simulink library "inp"  (R2021b)
settings: Solver=VariableStepAuto  StartTime=0.0  StopTime=10.0  RelTol=1e-3
undefined symbols (not defined in the file): C_TASK_5MS_S, FALSE, KINP_AcoreReadyToSlp_flg_ovrdflg, KINP_AcoreReadyToSlp_flg_ovrdval, KINP_AllowMovThd_OTA_enum_ovrdflg, KINP_AllowMovThd_OTA_enum_ovrdval, KINP_APSAngleTarget_Deg_ovrdflg, KINP_APSAngleTarget_Deg_ovrdval, KINP_APSDecReq_mps2_ovrdflg, KINP_APSDecReq_mps2_ovrdval, KINP_APSDecReqA_flg_ovrdflg, KINP_APSDecReqA_flg_ovrdval, KINP_APSDFLL_cm_ovrdflg, KINP_APSDFLL_cm_ovrdval, KINP_APSDFLR_cm_ovrdflg, KINP_APSDFLR_cm_ovrdval, KINP_APSDRLL_cm_ovrdflg, KINP_APSDRLL_cm_ovrdval, KINP_APSDRLR_cm_ovrdflg, KINP_APSDRLR_cm_ovrdval, KINP_APSExitCondition_enum_ovrdflg, KINP_APSExitCondition_enum_ovrdval, KINP_APSHWVer_enum_ovrdflg, KINP_APSHWVer_enum_ovrdval, KINP_APSProgressPCT_pct_ovrdflg, KINP_APSProgressPCT_pct_ovrdval, KINP_APSReq_enum_ovrdflg, KINP_APSReq_enum_ovrdval, KINP_APSRQDisplay_enum_ovrdflg, KINP_APSRQDisplay_enum_ovrdval, KINP_APSRqEPASCtrl_flg_ovrdflg, KINP_APSRqEPASCtrl_flg_ovrdval, KINP_APSShiftPosnReq_enum_ovrdval, KINP_APSShiftPosnReq_enum_ovrflg, KINP_APSSpeedCMD_kph_ovrdval, KINP_APSSpeedCMD_kph_ovrflg, KINP_APSStaSystem_enum_ovrdflg, KINP_APSStaSystem_enum_ovrdval, KINP_APSSWVer_enum_ovrdflg, KINP_APSSWVer_enum_ovrdval, KINP_APSVMCReqA_flg_ovrdval, KINP_APSVMCReqA_flg_ovrflg, KINP_APSVRqEPASCtrl_flg_ovrdflg, KINP_APSVRqEPASCtrl_flg_ovrdval, KINP_AuxBattVolmV_mV_ovrdflg, KINP_AuxBattVolmV_mV_ovrdval, KINP_CAASSta_enum_ovrdflg, KINP_CAASSta_enum_ovrdval, KINP_CAASVMCReqA_flg_ovrdval, KINP_CAASVMCReqA_flg_ovrflg, KINP_Chime_enum_ovrdflg, KINP_Chime_enum_ovrdval, KINP_ClearDTCcmd_flg_ovrdflg, KINP_ClearDTCcmd_flg_ovrdval, KINP_EvccAplusPwrUpReq_flg_ovrdflg, KINP_EvccAplusPwrUpReq_flg_ovrdval, KINP_LFID_raw_ovrdval, KINP_LFID_raw_ovrflg, KINP_LRID_raw_ovrdval, KINP_MemOffsetAccX_raw16_ovrdflg ... (+118)
libraries: FVT_lib x595, hcu_lib x1
(part 8 of 27)

== system inp/INP/GPIO/Digital ==
  BHAL_outputs : Inport
  BrakeLampSW : FVT_lib/inp/di_signal_template  SystemSampleTime=-1  VariantActivationTime=update diagram  Latency=0  AutoFrameSizeCalculation=off
      link override debdec: Value=KINP_BrakeLampSW_flg_debdec
      link override debinc: Value=KINP_BrakeLampSW_flg_debinc
      link override deblim: Value=KINP_BrakeLampSW_flg_deblim
      link override inverse: Value=KINP_BrakeLampSW_flg_inverse
      link override ovrdflg: Value=KINP_BrakeLampSW_flg_ovrdflg
      link override ovrdval: Value=KINP_BrakeLampSW_flg_ovrdval
      link override srvcflg: Value=KINP_BrakeLampSW_flg_srvcflg
      link override srvcval: Value=KINP_BrakeLampSW_flg_srvcval
  BrakeSWGPIO : FVT_lib/inp/di_signal_template  SystemSampleTime=-1  VariantActivationTime=update diagram  Latency=0  AutoFrameSizeCalculation=off
      link override debdec: Value=KINP_BrakeSWGPIO_flg_debdec
      link override debinc: Value=KINP_BrakeSWGPIO_flg_debinc
      link override deblim: Value=KINP_BrakeSWGPIO_flg_deblim
      link override inverse: Value=KINP_BrakeSWGPIO_flg_inverse
      link override ovrdflg: Value=KINP_BrakeSWGPIO_flg_ovrdflg
      link override ovrdval: Value=KINP_BrakeSWGPIO_flg_ovrdval
      link override srvcflg: Value=KINP_BrakeSWGPIO_flg_srvcflg
      link override srvcval: Value=KINP_BrakeSWGPIO_flg_srvcval
  CentralDoorLockSW : FVT_lib/inp/di_signal_template  SystemSampleTime=-1  VariantActivationTime=update diagram  Latency=0  AutoFrameSizeCalculation=off
      link override debdec: Value=KINP_CentralDoorLockSW_flg_debdec
      link override debinc: Value=KINP_CentralDoorLockSW_flg_debinc
      link override deblim: Value=KINP_CentralDoorLockSW_flg_deblim
      link override inverse: Value=KINP_CentralDoorLockSW_flg_inverse
      link override ovrdflg: Value=KINP_CentralDoorLockSW_flg_ovrdflg
      link override ovrdval: Value=KINP_CentralDoorLockSW_flg_ovrdval
      link override srvcflg: Value=KINP_CentralDoorLockSW_flg_srvcflg
      link override srvcval: Value=KINP_CentralDoorLockSW_flg_srvcval
  CrashSignalGPIO : FVT_lib/inp/di_signal_template  SystemSampleTime=-1  VariantActivationTime=update diagram  Latency=0  AutoFrameSizeCalculation=off
      link override debdec: Value=KINP_CrashSignalGPIO_flg_debdec
      link override debinc: Value=KINP_CrashSignalGPIO_flg_debinc
      link override deblim: Value=KINP_CrashSignalGPIO_flg_deblim
      link override inverse: Value=KINP_CrashSignalGPIO_flg_inverse
      link override ovrdflg: Value=KINP_CrashSignalGPIO_flg_ovrdflg
      link override ovrdval: Value=KINP_CrashSignalGPIO_flg_ovrdval
      link override srvcflg: Value=KINP_CrashSignalGPIO_flg_srvcflg
      link override srvcval: Value=KINP_CrashSignalGPIO_flg_srvcval
  DrDoorSW : FVT_lib/inp/di_signal_template  SystemSampleTime=-1  VariantActivationTime=update diagram  Latency=0  AutoFrameSizeCalculation=off
      link override debdec: Value=KINP_DrDoorSW_flg_debdec
      link override debinc: Value=KINP_DrDoorSW_flg_debinc
      link override deblim: Value=KINP_DrDoorSW_flg_deblim
      link override inverse: Value=KINP_DrDoorSW_flg_inverse
      link override ovrdflg: Value=KINP_DrDoorSW_flg_ovrdflg
      link override ovrdval: Value=KINP_DrDoorSW_flg_ovrdval
      link override srvcflg: Value=KINP_DrDoorSW_flg_srvcflg
      link override srvcval: Value=KINP_DrDoorSW_flg_srvcval
  HazardSW : FVT_lib/inp/di_signal_template  SystemSampleTime=-1  VariantActivationTime=update diagram  Latency=0  AutoFrameSizeCalculation=off
      link override debdec: Value=KINP_HazardSW_flg_debdec
      link override debinc: Value=KINP_HazardSW_flg_debinc
      link override deblim: Value=KINP_HazardSW_flg_deblim
      link override inverse: Value=KINP_HazardSW_flg_inverse
      link override ovrdflg: Value=KINP_HazardSW_flg_ovrdflg
      link override ovrdval: Value=KINP_HazardSW_flg_ovrdval
      link override srvcflg: Value=KINP_HazardSW_flg_srvcflg
      link override srvcval: Value=KINP_HazardSW_flg_srvcval
  HoodSW : FVT_lib/inp/di_signal_template  SystemSampleTime=-1  VariantActivationTime=update diagram  Latency=0  AutoFrameSizeCalculation=off
      link override debdec: Value=KINP_HoodSW_flg_debdec
      link override debinc: Value=KINP_HoodSW_flg_debinc
      link override deblim: Value=KINP_HoodSW_flg_deblim
      link override inverse: Value=KINP_HoodSW_flg_inverse
      link override ovrdflg: Value=KINP_HoodSW_flg_ovrdflg
      link override ovrdval: Value=KINP_HoodSW_flg_ovrdval
      link override srvcflg: Value=KINP_HoodSW_flg_srvcflg
      link override srvcval: Value=KINP_HoodSW_flg_srvcval
  PsDoorSW : FVT_lib/inp/di_signal_template  SystemSampleTime=-1  VariantActivationTime=update diagram  Latency=0  AutoFrameSizeCalculation=off
      link override debdec: Value=KINP_PsDoorSW_flg_debdec
      link override debinc: Value=KINP_PsDoorSW_flg_debinc
      link override deblim: Value=KINP_PsDoorSW_flg_deblim
      link override inverse: Value=KINP_PsDoorSW_flg_inverse
      link override ovrdflg: Value=KINP_PsDoorSW_flg_ovrdflg
      link override ovrdval: Value=KINP_PsDoorSW_flg_ovrdval
      link override srvcflg: Value=KINP_PsDoorSW_flg_srvcflg
      link override srvcval: Value=KINP_PsDoorSW_flg_srvcval
  RLDoorSW : FVT_lib/inp/di_signal_template  SystemSampleTime=-1  VariantActivationTime=update diagram  Latency=0  AutoFrameSizeCalculation=off
      link override debdec: Value=KINP_RLDoorSW_flg_debdec
      link override debinc: Value=KINP_RLDoorSW_flg_debinc
      link override deblim: Value=KINP_RLDoorSW_flg_deblim
      link override inverse: Value=KINP_RLDoorSW_flg_inverse
      link override ovrdflg: Value=KINP_RLDoorSW_flg_ovrdflg
      link override ovrdval: Value=KINP_RLDoorSW_flg_ovrdval
      link override srvcflg: Value=KINP_RLDoorSW_flg_srvcflg
      link override srvcval: Value=KINP_RLDoorSW_flg_srvcval
  RRDoorSW : FVT_lib/inp/di_signal_template  SystemSampleTime=-1  VariantActivationTime=update diagram  Latency=0  AutoFrameSizeCalculation=off
      link override debdec: Value=KINP_RRDoorSW_flg_debdec
      link override debinc: Value=KINP_RRDoorSW_flg_debinc
      link override deblim: Value=KINP_RRDoorSW_flg_deblim
      link override inverse: Value=KINP_RRDoorSW_flg_inverse
      link override ovrdflg: Value=KINP_RRDoorSW_flg_ovrdflg
      link override ovrdval: Value=KINP_RRDoorSW_flg_ovrdval
      link override srvcflg: Value=KINP_RRDoorSW_flg_srvcflg
      link override srvcval: Value=KINP_RRDoorSW_flg_srvcval
  SeatSW : FVT_lib/inp/di_signal_template  SystemSampleTime=-1  VariantActivationTime=update diagram  Latency=0  AutoFrameSizeCalculation=off
      link override debdec: Value=KINP_SeatSW_flg_debdec
      link override debinc: Value=KINP_SeatSW_flg_debinc
      link override deblim: Value=KINP_SeatSW_flg_deblim
      link override inverse: Value=KINP_SeatSW_flg_inverse
      link override ovrdflg: Value=KINP_SeatSW_flg_ovrdflg
      link override ovrdval: Value=KINP_SeatSW_flg_ovrdval
      link override srvcflg: Value=KINP_SeatSW_flg_srvcflg
      link override srvcval: Value=KINP_SeatSW_flg_srvcval
  TailgateSW : FVT_lib/inp/di_signal_template  SystemSampleTime=-1  VariantActivationTime=update diagram  Latency=0  AutoFrameSizeCalculation=off
      link override debdec: Value=KINP_TailgateSW_flg_debdec
      link override debinc: Value=KINP_TailgateSW_flg_debinc
      link override deblim: Value=KINP_TailgateSW_flg_deblim
      link override inverse: Value=KINP_TailgateSW_flg_inverse
      link override ovrdflg: Value=KINP_TailgateSW_flg_ovrdflg
      link override ovrdval: Value=KINP_TailgateSW_flg_ovrdval
      link override srvcflg: Value=KINP_TailgateSW_flg_srvcflg
      link override srvcval: Value=KINP_TailgateSW_flg_srvcval
  TrunkHanSW : FVT_lib/inp/di_signal_template  SystemSampleTime=-1  VariantActivationTime=update diagram  Latency=0  AutoFrameSizeCalculation=off
      link override debdec: Value=KINP_TrunkHanSW_flg_debdec
      link override debinc: Value=KINP_TrunkHanSW_flg_debinc
      link override deblim: Value=KINP_TrunkHanSW_flg_deblim
      link override inverse: Value=KINP_TrunkHanSW_flg_inverse
      link override ovrdflg: Value=KINP_TrunkHanSW_flg_ovrdflg
      link override ovrdval: Value=KINP_TrunkHanSW_flg_ovrdval
      link override srvcflg: Value=KINP_TrunkHanSW_flg_srvcflg
      link override srvcval: Value=KINP_TrunkHanSW_flg_srvcval
  slr_VINP_BrakeLampSW_flg : BusSelector  OutputSignals=VHAL_BrakeLampSW_flg
  slr_VINP_BrakeSWGPIO_flg : BusSelector  OutputSignals=VHAL_BrakeSWGPIO_flg
  slr_VINP_CentralDoorLockSW_flg : BusSelector  OutputSignals=VHAL_CentralDoorLockSW_flg
  slr_VINP_CrashSignalGPIO_flg : BusSelector  OutputSignals=VHAL_CrashSignalGPIO_flg
  slr_VINP_DrDoorSW_flg : BusSelector  OutputSignals=VHAL_DrDoorSW_flg
  slr_VINP_HazardSW_flg : BusSelector  OutputSignals=VHAL_HazardSW_flg
  slr_VINP_HoodSW_flg : BusSelector  OutputSignals=VHAL_HoodSW_flg
  slr_VINP_PsDoorSW_flg : BusSelector  OutputSignals=VHAL_PsDoorSW_flg
  slr_VINP_RLDoorSW_flg : BusSelector  OutputSignals=VHAL_RLDoorSW_flg
  slr_VINP_RRDoorSW_flg : BusSelector  OutputSignals=VHAL_RRDoorSW_flg
  slr_VINP_SeatSW_flg : BusSelector  OutputSignals=VHAL_SeatSW_flg
  slr_VINP_TailgateSW_flg : BusSelector  OutputSignals=VHAL_TailgateSW_flg
  slr_VINP_TrunkHanSW_flg : BusSelector  OutputSignals=VHAL_TrunkHanSW_flg
  VINP_BrakeSWGPIO_flg : Outport
  VINP_HoodSW_flg : Outport  Port=2
  VINP_TailgateSW_flg : Outport  Port=3
  VINP_DrDoorSW_flg : Outport  Port=4
  VINP_PsDoorSW_flg : Outport  Port=5
  VINP_RRDoorSW_flg : Outport  Port=6
  VINP_RLDoorSW_flg : Outport  Port=7
  VINP_CentralDoorLockSW_flg : Outport  Port=8
  VINP_HazardSW_flg : Outport  Port=9
  VINP_BrakeLampSW_flg : Outport  Port=10
  VINP_TrunkHanSW_flg : Outport  Port=11
  VINP_SeatSW_flg : Outport  Port=12
  VINP_CrashSignalGPIO_flg : Outport  Port=13
  wires:
  BHAL_outputs/1 -> [BHAL_outputs]
  BrakeSWGPIO/1 -> VINP_BrakeSWGPIO_flg/1  "VINP_BrakeSWGPIO_flg"
  [BHAL_outputs] -> slr_VINP_BrakeSWGPIO_flg/1
  slr_VINP_BrakeSWGPIO_flg/1 -> BrakeSWGPIO/1  "<VHAL_BrakeSWGPIO_flg>"
  HoodSW/1 -> VINP_HoodSW_flg/1  "VINP_HoodSW_flg"
  [BHAL_outputs] -> slr_VINP_HoodSW_flg/1
  slr_VINP_HoodSW_flg/1 -> HoodSW/1  "<VHAL_HoodSW_flg>"
  TailgateSW/1 -> VINP_TailgateSW_flg/1  "VINP_TailgateSW_flg"
  [BHAL_outputs] -> slr_VINP_TailgateSW_flg/1
  slr_VINP_TailgateSW_flg/1 -> TailgateSW/1  "<VHAL_TailgateSW_flg>"
  DrDoorSW/1 -> VINP_DrDoorSW_flg/1  "VINP_DrDoorSW_flg"
  [BHAL_outputs] -> slr_VINP_DrDoorSW_flg/1
  slr_VINP_DrDoorSW_flg/1 -> DrDoorSW/1  "<VHAL_DrDoorSW_flg>"
  PsDoorSW/1 -> VINP_PsDoorSW_flg/1  "VINP_PsDoorSW_flg"
  [BHAL_outputs] -> slr_VINP_PsDoorSW_flg/1
  slr_VINP_PsDoorSW_flg/1 -> PsDoorSW/1  "<VHAL_PsDoorSW_flg>"
  RRDoorSW/1 -> VINP_RRDoorSW_flg/1  "VINP_RRDoorSW_flg"
  [BHAL_outputs] -> slr_VINP_RRDoorSW_flg/1
  slr_VINP_RRDoorSW_flg/1 -> RRDoorSW/1  "<VHAL_RRDoorSW_flg>"
  RLDoorSW/1 -> VINP_RLDoorSW_flg/1  "VINP_RLDoorSW_flg"
  [BHAL_outputs] -> slr_VINP_RLDoorSW_flg/1
  slr_VINP_RLDoorSW_flg/1 -> RLDoorSW/1  "<VHAL_RLDoorSW_flg>"
  CentralDoorLockSW/1 -> VINP_CentralDoorLockSW_flg/1  "VINP_CentralDoorLockSW_flg"
  [BHAL_outputs] -> slr_VINP_CentralDoorLockSW_flg/1
  slr_VINP_CentralDoorLockSW_flg/1 -> CentralDoorLockSW/1  "<VHAL_CentralDoorLockSW_flg>"
  HazardSW/1 -> VINP_HazardSW_flg/1  "VINP_HazardSW_flg"
  [BHAL_outputs] -> slr_VINP_HazardSW_flg/1
  slr_VINP_HazardSW_flg/1 -> HazardSW/1  "<VHAL_HazardSW_flg>"
  BrakeLampSW/1 -> VINP_BrakeLampSW_flg/1  "VINP_BrakeLampSW_flg"
  [BHAL_outputs] -> slr_VINP_BrakeLampSW_flg/1
  slr_VINP_BrakeLampSW_flg/1 -> BrakeLampSW/1  "<VHAL_BrakeLampSW_flg>"
  TrunkHanSW/1 -> VINP_TrunkHanSW_flg/1  "VINP_TrunkHanSW_flg"
  [BHAL_outputs] -> slr_VINP_TrunkHanSW_flg/1
  slr_VINP_TrunkHanSW_flg/1 -> TrunkHanSW/1  "<VHAL_TrunkHanSW_flg>"
  SeatSW/1 -> VINP_SeatSW_flg/1  "VINP_SeatSW_flg"
  [BHAL_outputs] -> slr_VINP_SeatSW_flg/1
  slr_VINP_SeatSW_flg/1 -> SeatSW/1  "<VHAL_SeatSW_flg>"
  [BHAL_outputs] -> slr_VINP_CrashSignalGPIO_flg/1
  slr_VINP_CrashSignalGPIO_flg/1 -> CrashSignalGPIO/1  "<VHAL_CrashSignalGPIO_flg>"
  CrashSignalGPIO/1 -> VINP_CrashSignalGPIO_flg/1  "VINP_CrashSignalGPIO_flg"

== system inp/INP/IMU/Subsystem1 ==
  In1 : Inport
  Constant : Constant  Value=KINP_MemOffsetGyroY_raw16_ovrdval
  Constant1 : Constant  Value=KINP_MemOffsetGyroY_raw16_ovrdflg
  Switch : Switch  Criteria=u2 ~= 0
  Out1 : Outport
  wires:
  Switch/1 -> Out1/1
  Constant/1 -> Switch/1
  Constant1/1 -> Switch/2
  In1/1 -> Switch/3

== system inp/INP/IMU/Subsystem10 ==
  In1 : Inport
  Constant : Constant  Value=KINP_SensingAccZ_raw16_ovrdval
  Constant1 : Constant  Value=KINP_SensingAccZ_raw16_ovrdflg
  Switch : Switch  Criteria=u2 ~= 0
  Out1 : Outport
  wires:
  Constant1/1 -> Switch/2
  Constant/1 -> Switch/1
  Switch/1 -> Out1/1
  In1/1 -> Switch/3

== system inp/INP/IMU/Subsystem11 ==
  In1 : Inport
  Constant : Constant  Value=KINP_SensingAccY_raw16_ovrdval
  Constant1 : Constant  Value=KINP_SensingAccY_raw16_ovrdflg
  Switch : Switch  Criteria=u2 ~= 0
  Out1 : Outport
  wires:
  Switch/1 -> Out1/1
  Constant/1 -> Switch/1
  Constant1/1 -> Switch/2
  In1/1 -> Switch/3

== system inp/INP/IMU/Subsystem15 ==
  In1 : Inport
  Constant : Constant  Value=KINP_MemOffsetGyroX_raw16_ovrdval
  Constant1 : Constant  Value=KINP_MemOffsetGyroX_raw16_ovrdflg
  Switch : Switch  Criteria=u2 ~= 0
  Out1 : Outport
  wires:
  Constant1/1 -> Switch/2
  Constant/1 -> Switch/1
  Switch/1 -> Out1/1
  In1/1 -> Switch/3

== system inp/INP/IMU/Subsystem2 ==
  In1 : Inport
  Constant : Constant  Value=KINP_MemOffsetAccX_raw16_ovrdval
  Constant1 : Constant  Value=KINP_MemOffsetAccX_raw16_ovrdflg
  Switch : Switch  Criteria=u2 ~= 0
  Out1 : Outport
  wires:
  Constant1/1 -> Switch/2
  Constant/1 -> Switch/1
  Switch/1 -> Out1/1
  In1/1 -> Switch/3

== system inp/INP/IMU/Subsystem3 ==
  In1 : Inport
  Constant : Constant  Value=KINP_MemOffsetGyroZ_raw16_ovrdval
  Constant1 : Constant  Value=KINP_MemOffsetGyroZ_raw16_ovrdflg
  Switch : Switch  Criteria=u2 ~= 0
  Out1 : Outport
  wires:
  Switch/1 -> Out1/1
  Constant/1 -> Switch/1
  Constant1/1 -> Switch/2
  In1/1 -> Switch/3

== system inp/INP/IMU/Subsystem4 ==
  In1 : Inport
  Constant : Constant  Value=KINP_MemOffsetAccZ_raw16_ovrdval
  Constant1 : Constant  Value=KINP_MemOffsetAccZ_raw16_ovrdflg
  Switch : Switch  Criteria=u2 ~= 0
  Out1 : Outport
  wires:
  Switch/1 -> Out1/1
  Constant/1 -> Switch/1
  Constant1/1 -> Switch/2
  In1/1 -> Switch/3

== system inp/INP/IMU/Subsystem5 ==
  In1 : Inport
  Constant : Constant  Value=KINP_MemOffsetAccY_raw16_ovrdval
  Constant1 : Constant  Value=KINP_MemOffsetAccY_raw16_ovrdflg
  Switch : Switch  Criteria=u2 ~= 0
  Out1 : Outport
  wires:
  Constant1/1 -> Switch/2
  Constant/1 -> Switch/1
  Switch/1 -> Out1/1
  In1/1 -> Switch/3

== system inp/INP/IMU/Subsystem6 ==
  In1 : Inport
  Constant : Constant  Value=KINP_SensingGyroY_raw16_ovrdval
  Constant1 : Constant  Value=KINP_SensingGyroY_raw16_ovrdflg
  Switch : Switch  Criteria=u2 ~= 0
  Out1 : Outport
  wires:
  Constant1/1 -> Switch/2
  Constant/1 -> Switch/1
  Switch/1 -> Out1/1
  In1/1 -> Switch/3

== system inp/INP/IMU/Subsystem7 ==
  In1 : Inport
  Constant : Constant  Value=KINP_SensingGyroX_raw16_ovrdval
  Constant1 : Constant  Value=KINP_SensingGyroX_raw16_ovrdflg
  Switch : Switch  Criteria=u2 ~= 0
  Out1 : Outport
  wires:
  Switch/1 -> Out1/1
  Constant/1 -> Switch/1
  Constant1/1 -> Switch/2
  In1/1 -> Switch/3

== system inp/INP/IMU/Subsystem8 ==
  In1 : Inport
  Constant : Constant  Value=KINP_SensingAccX_raw16_ovrdval
  Constant1 : Constant  Value=KINP_SensingAccX_raw16_ovrdflg
  Switch : Switch  Criteria=u2 ~= 0
  Out1 : Outport
  wires:
  Switch/1 -> Out1/1
  Constant/1 -> Switch/1
  Constant1/1 -> Switch/2
  In1/1 -> Switch/3

== system inp/INP/IMU/Subsystem9 ==
  In1 : Inport
  Constant : Constant  Value=KINP_SensingGyroZ_raw16_ovrdval
  Constant1 : Constant  Value=KINP_SensingGyroZ_raw16_ovrdflg
  Switch : Switch  Criteria=u2 ~= 0
  Out1 : Outport
  wires:
  Constant1/1 -> Switch/2
  Constant/1 -> Switch/1
  Switch/1 -> Out1/1
  In1/1 -> Switch/3

== system inp/INP/SYS/Subsystem ==
  In1 : Inport
  Constant : Constant  Value=KINP_AuxBattVolmV_mV_ovrdflg
  Constant1 : Constant  Value=KINP_AuxBattVolmV_mV_ovrdval
  Switch : Switch  Criteria=u2 > Threshold
  Out1 : Outport
  wires:
  Constant1/1 -> Switch/1
  Constant/1 -> Switch/2
  In1/1 -> Switch/3
  Switch/1 -> Out1/1

== system inp/INP/SYS/Subsystem1 ==
  In1 : Inport
  Constant : Constant  Value=KINP_NetworkReqCalled_flg_ovrdflg
  Constant1 : Constant  Value=KINP_NetworkReqCalled_flg_ovrdval
  Switch : Switch  Criteria=u2 > Threshold
  Out1 : Outport
  wires:
  Constant1/1 -> Switch/1
  Constant/1 -> Switch/2
  In1/1 -> Switch/3
  Switch/1 -> Out1/1

== system inp/INP/SYS/Subsystem2 ==
  In1 : Inport
  Constant : Constant  Value=KINP_Pedal1Ref5V_V_ovrdflg
  Constant1 : Constant  Value=KINP_Pedal1Ref5V_V_ovrdval
  Switch : Switch  Criteria=u2 > Threshold
  Out1 : Outport
  wires:
  Switch/1 -> Out1/1
  In1/1 -> Switch/3
  Constant/1 -> Switch/2
  Constant1/1 -> Switch/1

== system inp/INP/SYS/Subsystem3 ==
  In1 : Inport
  Constant : Constant  Value=KINP_Pedal2Ref5V_V_ovrdflg
  Constant1 : Constant  Value=KINP_Pedal2Ref5V_V_ovrdval
  Switch : Switch  Criteria=u2 > Threshold
  Out1 : Outport
  wires:
  Constant1/1 -> Switch/1
  Constant/1 -> Switch/2
  In1/1 -> Switch/3
  Switch/1 -> Out1/1

== system inp/INP/SYS/Subsystem4 ==
  In1 : Inport
  Constant : Constant  Value=KINP_PwrReq_OTA_enum_ovrdval
  Constant1 : Constant  Value=KINP_PwrReq_OTA_enum_ovrdflg
  Switch : Switch  Criteria=u2 ~= 0
  Out1 : Outport
  wires:
  Constant1/1 -> Switch/2
  Constant/1 -> Switch/1
  In1/1 -> Switch/3
  Switch/1 -> Out1/1

== system inp/INP/SYS/Subsystem5 ==
  In1 : Inport
  Constant : Constant  Value=KINP_AllowMovThd_OTA_enum_ovrdval
  Constant1 : Constant  Value=KINP_AllowMovThd_OTA_enum_ovrdflg
  Switch : Switch  Criteria=u2 ~= 0
  Out1 : Outport
  wires:
  Switch/1 -> Out1/1
  In1/1 -> Switch/3
  Constant/1 -> Switch/1
  Constant1/1 -> Switch/2

== system inp/INP/SYS/Subsystem6 ==
  In1 : Inport
  Constant : Constant  Value=KINP_EvccAplusPwrUpReq_flg_ovrdval
  Constant1 : Constant  Value=KINP_EvccAplusPwrUpReq_flg_ovrdflg
  Switch : Switch  Criteria=u2 ~= 0
  Out1 : Outport
  wires:
  Constant1/1 -> Switch/2
  Constant/1 -> Switch/1
  In1/1 -> Switch/3
  Switch/1 -> Out1/1

== system inp/INP/SYS/Subsystem7 ==
  In1 : Inport
  Constant : Constant  Value=KINP_AcoreReadyToSlp_flg_ovrdval
  Constant1 : Constant  Value=KINP_AcoreReadyToSlp_flg_ovrdflg
  Switch : Switch  Criteria=u2 ~= 0
  Out1 : Outport
  wires:
  Switch/1 -> Out1/1
  In1/1 -> Switch/3
  Constant/1 -> Switch/1
  Constant1/1 -> Switch/2

== system inp/INP/Subsystem/Subsystem13 ==
  In1 : Inport
  Constant : Constant  Value=KINP_ClearDTCcmd_flg_ovrdval
  Constant1 : Constant  Value=KINP_ClearDTCcmd_flg_ovrdflg
  Switch : Switch  Criteria=u2 ~= 0
  Out1 : Outport
  wires:
  Constant1/1 -> Switch/2
  Constant/1 -> Switch/1
  Switch/1 -> Out1/1
  In1/1 -> Switch/3

== system inp/INP/TPMS/Subsystem ==
  In1 : Inport
  Constant : Constant  Value=KINP_TPMSDataIn_flg_ovrdval
  Constant1 : Constant  Value=KINP_TPMSDataIn_flg_ovrdflg
  Switch : Switch  Criteria=u2 ~= 0
  Out1 : Outport
  wires:
  Switch/1 -> Out1/1
  In1/1 -> Switch/3
  Constant/1 -> Switch/1
  Constant1/1 -> Switch/2

== system inp/INP/TPMS/Subsystem1 ==
  In1 : Inport
  Constant : Constant  Value=KINP_TPMSID_raw_ovrdflg
  Constant1 : Constant  Value=KINP_TPMSID_raw_ovrdval
  Switch : Switch  Criteria=u2 ~= 0
  Out1 : Outport
  wires:
  Constant/1 -> Switch/2
  Constant1/1 -> Switch/1
  Switch/1 -> Out1/1
  In1/1 -> Switch/3

== system inp/INP/TPMS/Subsystem10 ==
  In1 : Inport
  Constant : Constant  Value=KINP_TPMSStorge_flg_ovrflg
  Constant1 : Constant  Value=KINP_TPMSStorge_flg_ovrdval
  Switch : Switch  Criteria=u2 ~= 0
  Out1 : Outport
  wires:
  Constant1/1 -> Switch/1
  Constant/1 -> Switch/2
  In1/1 -> Switch/3
  Switch/1 -> Out1/1

== system inp/INP/TPMS/Subsystem11 ==
  In1 : Inport
  Constant : Constant  Value=KINP_LFID_raw_ovrflg
  Constant1 : Constant  Value=KINP_LFID_raw_ovrdval
  Switch : Switch  Criteria=u2 ~= 0
  Out1 : Outport
  wires:
  Switch/1 -> Out1/1
  In1/1 -> Switch/3
  Constant/1 -> Switch/2
  Constant1/1 -> Switch/1

== system inp/INP/TPMS/Subsystem12 ==
  In1 : Inport
  Constant : Constant  Value=KINP_RFID_raw_ovrdval
  Constant1 : Constant  Value=KINP_RFID_raw_ovrdval
  Switch : Switch  Criteria=u2 ~= 0
  Out1 : Outport
  wires:
  Constant1/1 -> Switch/1
  Constant/1 -> Switch/2
  In1/1 -> Switch/3
  Switch/1 -> Out1/1

== system inp/INP/TPMS/Subsystem13 ==
  In1 : Inport
  Constant : Constant  Value=KINP_LRID_raw_ovrdval
  Constant1 : Constant  Value=KINP_LRID_raw_ovrdval
  Switch : Switch  Criteria=u2 ~= 0
  Out1 : Outport
  wires:
  Switch/1 -> Out1/1
  In1/1 -> Switch/3
  Constant/1 -> Switch/2
  Constant1/1 -> Switch/1

== system inp/INP/TPMS/Subsystem14 ==
  In1 : Inport
  Constant : Constant  Value=KINP_RRID_raw_ovrdval
  Constant1 : Constant  Value=KINP_RRID_raw_ovrdval
  Switch : Switch  Criteria=u2 ~= 0
  Out1 : Outport
  wires:
  Constant1/1 -> Switch/1
  Constant/1 -> Switch/2
  In1/1 -> Switch/3
  Switch/1 -> Out1/1

== system inp/INP/TPMS/Subsystem2 ==
  In1 : Inport
  Constant : Constant  Value=KINP_TPMSPressure_raw_ovrdflg
  Constant1 : Constant  Value=KINP_TPMSPressure_raw_ovrdval
  Switch : Switch  Criteria=u2 ~= 0
  Out1 : Outport
  wires:
  Constant/1 -> Switch/2
  Constant1/1 -> Switch/1
  Switch/1 -> Out1/1
  In1/1 -> Switch/3

== system inp/INP/TPMS/Subsystem3 ==
  In1 : Inport
  Constant : Constant  Value=KINP_TPMSTemp_raw_ovrdflg
  Constant1 : Constant  Value=KINP_TPMSTemp_raw_ovrdval
  Switch : Switch  Criteria=u2 ~= 0
  Out1 : Outport
  wires:
  Constant/1 -> Switch/2
  Constant1/1 -> Switch/1
  Switch/1 -> Out1/1
  In1/1 -> Switch/3

== system inp/INP/TPMS/Subsystem4 ==
  In1 : Inport
  Constant : Constant  Value=KINP_TPMSSta_enum_ovrdflg
  Constant1 : Constant  Value=KINP_TPMSSta_enum_ovrdval
  Switch : Switch  Criteria=u2 ~= 0
  Out1 : Outport
  wires:
  Constant/1 -> Switch/2
  Constant1/1 -> Switch/1
  Switch/1 -> Out1/1
  In1/1 -> Switch/3

== system inp/INP/TPMS/Subsystem5 ==
  In1 : Inport
  Constant : Constant  Value=KINP_TPMSPressureMi_raw_ovrdflg
  Constant1 : Constant  Value=KINP_TPMSPressureMi_raw_ovrdval
  Switch : Switch  Criteria=u2 ~= 0
  Out1 : Outport
  wires:
  Constant/1 -> Switch/2
  Constant1/1 -> Switch/1
  Switch/1 -> Out1/1
  In1/1 -> Switch/3

== system inp/INP/TPMS/Subsystem6 ==
  In1 : Inport
  Constant : Constant  Value=KINP_TPMSCRC_crc_ovrdflg
  Constant1 : Constant  Value=KINP_TPMSCRC_crc_ovrdval
  Switch : Switch  Criteria=u2 ~= 0
  Out1 : Outport
  wires:
  Constant/1 -> Switch/2
  Constant1/1 -> Switch/1
  Switch/1 -> Out1/1
  In1/1 -> Switch/3

== system inp/INP/TPMS/Subsystem7 ==
  In1 : Inport
  Constant : Constant  Value=KINP_TPMSCRCCalc_crc_ovrdflg
  Constant1 : Constant  Value=KINP_TPMSCRCCalc_crc_ovrdval
  Switch : Switch  Criteria=u2 ~= 0
  Out1 : Outport
  wires:
  Constant/1 -> Switch/2
  Constant1/1 -> Switch/1
  Switch/1 -> Out1/1
  In1/1 -> Switch/3

== system inp/INP/TPMS/Subsystem8 ==
  In1 : Inport
  Constant : Constant  Value=KINP_TPMSFAT_flg_ovrflg
  Constant1 : Constant  Value=KINP_TPMSFAT_flg_ovrdval
  Switch : Switch  Criteria=u2 ~= 0
  Out1 : Outport
  wires:
  Switch/1 -> Out1/1
  In1/1 -> Switch/3
  Constant1/1 -> Switch/1
  Constant/1 -> Switch/2

== system inp/INP/TPMS/Subsystem9 ==
  In1 : Inport
  Constant : Constant  Value=KINP_TPMSBattLow_flg_ovrflg
  Constant1 : Constant  Value=KINP_TPMSBattLow_flg_ovrdval
  Switch : Switch  Criteria=u2 ~= 0
  Out1 : Outport
  wires:
  Switch/1 -> Out1/1
  In1/1 -> Switch/3
  Constant/1 -> Switch/2
  Constant1/1 -> Switch/1

== system inp/INP/CAN1/SignalCheck/ABM1 ==
  BHAL_outputs : Inport
  inp_CanValid_bus : Inport  Port=2
  ABM1CSErr : FVT_lib/inp/can_signal_template  SystemSampleTime=-1  VariantActivationTime=update diagram  Latency=0  AutoFrameSizeCalculation=off
      link override defval: Value=KINP_ABM1CSErr_flg_defval
      link override fftdec: Value=KINP_ABM1CSErr_flg_fftdec
      link override fftinc: Value=KINP_ABM1CSErr_flg_fftinc
      link override fftlim: Value=KINP_ABM1CSErr_flg_fftlim
      link override invalid: Value=KINP_ABM1CSErr_flg_invalid
      link override ovrdflg: Value=KINP_ABM1CSErr_flg_ovrdflg
      link override ovrdval: Value=KINP_ABM1CSErr_flg_ovrdval
      link override setvalid: Value=KINP_ABM1CSErr_flg_setvalid
      link override srvcflg: Value=KINP_ABM1CSErr_flg_srvcflg
      link override srvcval: Value=KINP_ABM1CSErr_flg_srvcval
  ABM1RCErr : FVT_lib/inp/can_signal_template  SystemSampleTime=-1  VariantActivationTime=update diagram  Latency=0  AutoFrameSizeCalculation=off
      link override defval: Value=KINP_ABM1RCErr_flg_defval
      link override fftdec: Value=KINP_ABM1RCErr_flg_fftdec
      link override fftinc: Value=KINP_ABM1RCErr_flg_fftinc
      link override fftlim: Value=KINP_ABM1RCErr_flg_fftlim
      link override invalid: Value=KINP_ABM1RCErr_flg_invalid
      link override ovrdflg: Value=KINP_ABM1RCErr_flg_ovrdflg
      link override ovrdval: Value=KINP_ABM1RCErr_flg_ovrdval
      link override setvalid: Value=KINP_ABM1RCErr_flg_setvalid
      link override srvcflg: Value=KINP_ABM1RCErr_flg_srvcflg
      link override srvcval: Value=KINP_ABM1RCErr_flg_srvcval
  AirBagFailCmd : FVT_lib/inp/can_signal_template  SystemSampleTime=-1  VariantActivationTime=update diagram  Latency=0  AutoFrameSizeCalculation=off
      link override defval: Value=KINP_AirBagFailCmd_flg_defval
      link override fftdec: Value=KINP_AirBagFailCmd_flg_fftdec
      link override fftinc: Value=KINP_AirBagFailCmd_flg_fftinc
      link override fftlim: Value=KINP_AirBagFailCmd_flg_fftlim
      link override invalid: Value=KINP_AirBagFailCmd_flg_invalid
      link override ovrdflg: Value=KINP_AirBagFailCmd_flg_ovrdflg
      link override ovrdval: Value=KINP_AirBagFailCmd_flg_ovrdval
      link override setvalid: Value=KINP_AirBagFailCmd_flg_setvalid
      link override srvcflg: Value=KINP_AirBagFailCmd_flg_srvcflg
      link override srvcval: Value=KINP_AirBagFailCmd_flg_srvcval
  ChecksumABM1 : FVT_lib/inp/can_signal_template  SystemSampleTime=-1  VariantActivationTime=update diagram  Latency=0  AutoFrameSizeCalculation=off
      link override defval: Value=KINP_ChecksumABM1_enum_defval
      link override fftdec: Value=KINP_ChecksumABM1_enum_fftdec
      link override fftinc: Value=KINP_ChecksumABM1_enum_fftinc
      link override fftlim: Value=KINP_ChecksumABM1_enum_fftlim
      link override invalid: Value=KINP_ChecksumABM1_enum_invalid
      link override ovrdflg: Value=KINP_ChecksumABM1_enum_ovrdflg
      link override ovrdval: Value=KINP_ChecksumABM1_enum_ovrdval
      link override setvalid: Value=KINP_ChecksumABM1_enum_setvalid
      link override srvcflg: Value=KINP_ChecksumABM1_enum_srvcflg
      link override srvcval: Value=KINP_ChecksumABM1_enum_srvcval
  CrashOutputSts : FVT_lib/inp/can_signal_template  SystemSampleTime=-1  VariantActivationTime=update diagram  Latency=0  AutoFrameSizeCalculation=off
      link override defval: Value=KINP_CrashOutputSts_enum_defval
      link override fftdec: Value=KINP_CrashOutputSts_enum_fftdec
      link override fftinc: Value=KINP_CrashOutputSts_enum_fftinc
      link override fftlim: Value=KINP_CrashOutputSts_enum_fftlim
      link override invalid: Value=KINP_CrashOutputSts_enum_invalid
      link override ovrdflg: Value=KINP_CrashOutputSts_enum_ovrdflg
      link override ovrdval: Value=KINP_CrashOutputSts_enum_ovrdval
      link override setvalid: Value=KINP_CrashOutputSts_enum_setvalid
      link override srvcflg: Value=KINP_CrashOutputSts_enum_srvcflg
      link override srvcval: Value=KINP_CrashOutputSts_enum_srvcval
  DriverSeatBeltCmd : FVT_lib/inp/can_signal_template  SystemSampleTime=-1  VariantActivationTime=update diagram  Latency=0  AutoFrameSizeCalculation=off
      link override defval: Value=KINP_DriverSeatBeltCmd_flg_defval
      link override fftdec: Value=KINP_DriverSeatBeltCmd_flg_fftdec
      link override fftinc: Value=KINP_DriverSeatBeltCmd_flg_fftinc
      link override fftlim: Value=KINP_DriverSeatBeltCmd_flg_fftlim
      link override invalid: Value=KINP_DriverSeatBeltCmd_flg_invalid
      link override ovrdflg: Value=KINP_DriverSeatBeltCmd_flg_ovrdflg
      link override ovrdval: Value=KINP_DriverSeatBeltCmd_flg_ovrdval
      link override setvalid: Value=KINP_DriverSeatBeltCmd_flg_setvalid
      link override srvcflg: Value=KINP_DriverSeatBeltCmd_flg_srvcflg
      link override srvcval: Value=KINP_DriverSeatBeltCmd_flg_srvcval
  LifeCountABM1 : FVT_lib/inp/can_signal_template  SystemSampleTime=-1  VariantActivationTime=update diagram  Latency=0  AutoFrameSizeCalculation=off
      link override defval: Value=KINP_LifeCountABM1_enum_defval
      link override fftdec: Value=KINP_LifeCountABM1_enum_fftdec
      link override fftinc: Value=KINP_LifeCountABM1_enum_fftinc
      link override fftlim: Value=KINP_LifeCountABM1_enum_fftlim
      link override invalid: Value=KINP_LifeCountABM1_enum_invalid
      link override ovrdflg: Value=KINP_LifeCountABM1_enum_ovrdflg
      link override ovrdval: Value=KINP_LifeCountABM1_enum_ovrdval
      link override setvalid: Value=KINP_LifeCountABM1_enum_setvalid
      link override srvcflg: Value=KINP_LifeCountABM1_enum_srvcflg
      link override srvcval: Value=KINP_LifeCountABM1_enum_srvcval
  PsngrSeatBeltCmd : FVT_lib/inp/can_signal_template  SystemSampleTime=-1  VariantActivationTime=update diagram  Latency=0  AutoFrameSizeCalculation=off
      link override defval: Value=KINP_PsngrSeatBeltCmd_flg_defval
      link override fftdec: Value=KINP_PsngrSeatBeltCmd_flg_fftdec
      link override fftinc: Value=KINP_PsngrSeatBeltCmd_flg_fftinc
      link override fftlim: Value=KINP_PsngrSeatBeltCmd_flg_fftlim
      link override invalid: Value=KINP_PsngrSeatBeltCmd_flg_invalid
      link override ovrdflg: Value=KINP_PsngrSeatBeltCmd_flg_ovrdflg
      link override ovrdval: Value=KINP_PsngrSeatBeltCmd_flg_ovrdval
      link override setvalid: Value=KINP_PsngrSeatBeltCmd_flg_setvalid
      link override srvcflg: Value=KINP_PsngrSeatBeltCmd_flg_srvcflg
      link override srvcval: Value=KINP_PsngrSeatBeltCmd_flg_srvcval
  RCenterSeatBeltCmd : FVT_lib/inp/can_signal_template  SystemSampleTime=-1  VariantActivationTime=update diagram  Latency=0  AutoFrameSizeCalculation=off
      link override defval: Value=KINP_RCenterSeatBeltCmd_flg_defval
      link override fftdec: Value=KINP_RCenterSeatBeltCmd_flg_fftdec
      link override fftinc: Value=KINP_RCenterSeatBeltCmd_flg_fftinc
      link override fftlim: Value=KINP_RCenterSeatBeltCmd_flg_fftlim
      link override invalid: Value=KINP_RCenterSeatBeltCmd_flg_invalid
      link override ovrdflg: Value=KINP_RCenterSeatBeltCmd_flg_ovrdflg
      link override ovrdval: Value=KINP_RCenterSeatBeltCmd_flg_ovrdval
      link override setvalid: Value=KINP_RCenterSeatBeltCmd_flg_setvalid
      link override srvcflg: Value=KINP_RCenterSeatBeltCmd_flg_srvcflg
      link override srvcval: Value=KINP_RCenterSeatBeltCmd_flg_srvcval
  RDriverSeatBeltCmd : FVT_lib/inp/can_signal_template  SystemSampleTime=-1  VariantActivationTime=update diagram  Latency=0  AutoFrameSizeCalculation=off
      link override defval: Value=KINP_RDriverSeatBeltCmd_flg_defval
      link override fftdec: Value=KINP_RDriverSeatBeltCmd_flg_fftdec
      link override fftinc: Value=KINP_RDriverSeatBeltCmd_flg_fftinc
      link override fftlim: Value=KINP_RDriverSeatBeltCmd_flg_fftlim
      link override invalid: Value=KINP_RDriverSeatBeltCmd_flg_invalid
      link override ovrdflg: Value=KINP_RDriverSeatBeltCmd_flg_ovrdflg
      link override ovrdval: Value=KINP_RDriverSeatBeltCmd_flg_ovrdval
      link override setvalid: Value=KINP_RDriverSeatBeltCmd_flg_setvalid
      link override srvcflg: Value=KINP_RDriverSeatBeltCmd_flg_srvcflg
      link override srvcval: Value=KINP_RDriverSeatBeltCmd_flg_srvcval
  RPsngrSeatBeltCmd : FVT_lib/inp/can_signal_template  SystemSampleTime=-1  VariantActivationTime=update diagram  Latency=0  AutoFrameSizeCalculation=off
      link override defval: Value=KINP_RPsngrSeatBeltCmd_flg_defval
      link override fftdec: Value=KINP_RPsngrSeatBeltCmd_flg_fftdec
      link override fftinc: Value=KINP_RPsngrSeatBeltCmd_flg_fftinc
      link override fftlim: Value=KINP_RPsngrSeatBeltCmd_flg_fftlim
      link override invalid: Value=KINP_RPsngrSeatBeltCmd_flg_invalid
      link override ovrdflg: Value=KINP_RPsngrSeatBeltCmd_flg_ovrdflg
      link override ovrdval: Value=KINP_RPsngrSeatBeltCmd_flg_ovrdval
      link override setvalid: Value=KINP_RPsngrSeatBeltCmd_flg_setvalid
      link override srvcflg: Value=KINP_RPsngrSeatBeltCmd_flg_srvcflg
      link override srvcval: Value=KINP_RPsngrSeatBeltCmd_flg_srvcval
  Terminator_{1..11} (11 alike) : Terminator
  True_VHAL_ABM1CSErr_flg : Constant  Value=TRUE  OutDataTypeStr=boolean
  True_VHAL_ABM1RCErr_flg : Constant  Value=TRUE  OutDataTypeStr=boolean
  True_VHAL_AirBagFailCmd_flg : Constant  Value=TRUE  OutDataTypeStr=boolean
  True_VHAL_ChecksumABM1_enum : Constant  Value=TRUE  OutDataTypeStr=boolean
  True_VHAL_CrashOutputSts_enum : Constant  Value=TRUE  OutDataTypeStr=boolean
  True_VHAL_DriverSeatBeltCmd_flg : Constant  Value=TRUE  OutDataTypeStr=boolean
  True_VHAL_LifeCountABM1_enum : Constant  Value=TRUE  OutDataTypeStr=boolean
  True_VHAL_PsngrSeatBeltCmd_flg : Constant  Value=TRUE  OutDataTypeStr=boolean
  True_VHAL_RCenterSeatBeltCmd_flg : Constant  Value=TRUE  OutDataTypeStr=boolean
  True_VHAL_RDriverSeatBeltCmd_flg : Constant  Value=TRUE  OutDataTypeStr=boolean
  True_VHAL_RPsngrSeatBeltCmd_flg : Constant  Value=TRUE  OutDataTypeStr=boolean
  slr1_{1..11} (11 alike) : BusSelector  OutputSignals=VINP_CANMsgValidABM1_flg
  slr_VHAL_ABM1CSErr_flg : BusSelector  OutputSignals=VHAL_ABM1CSErr_flg
  slr_VHAL_ABM1RCErr_flg : BusSelector  OutputSignals=VHAL_ABM1RCErr_flg
  slr_VHAL_AirBagFailCmd_flg : BusSelector  OutputSignals=VHAL_AirBagFailCmd_flg
  slr_VHAL_ChecksumABM1_enum : BusSelector  OutputSignals=VHAL_ChecksumABM1_enum
  slr_VHAL_CrashOutputSts_enum : BusSelector  OutputSignals=VHAL_CrashOutputSts_enum
  slr_VHAL_DriverSeatBeltCmd_flg : BusSelector  OutputSignals=VHAL_DriverSeatBeltCmd_flg
  slr_VHAL_LifeCountABM1_enum : BusSelector  OutputSignals=VHAL_LifeCountABM1_enum
  slr_VHAL_PsngrSeatBeltCmd_flg : BusSelector  OutputSignals=VHAL_PsngrSeatBeltCmd_flg
  slr_VHAL_RCenterSeatBeltCmd_flg : BusSelector  OutputSignals=VHAL_RCenterSeatBeltCmd_flg
  slr_VHAL_RDriverSeatBeltCmd_flg : BusSelector  OutputSignals=VHAL_RDriverSeatBeltCmd_flg
  slr_VHAL_RPsngrSeatBeltCmd_flg : BusSelector  OutputSignals=VHAL_RPsngrSeatBeltCmd_flg
  VINP_ABM1CSErr_flg : Outport
  VINP_ABM1RCErr_flg : Outport  Port=2
  VINP_AirBagFailCmd_flg : Outport  Port=3
  VINP_ChecksumABM1_enum : Outport  Port=4
  VINP_CrashOutputSts_enum : Outport  Port=5
  VINP_DriverSeatBeltCmd_flg : Outport  Port=6
  VINP_LifeCountABM1_enum : Outport  Port=7
  VINP_PsngrSeatBeltCmd_flg : Outport  Port=8
  VINP_RCenterSeatBeltCmd_flg : Outport  Port=9
  VINP_RDriverSeatBeltCmd_flg : Outport  Port=10
  VINP_RPsngrSeatBeltCmd_flg : Outport  Port=11
  wires:
  BHAL_outputs/1 -> [BHAL_outputs]
  inp_CanValid_bus/1 -> [inp_CanValid_bus]
  [BHAL_outputs] -> slr_VHAL_ABM1CSErr_flg/1
  slr_VHAL_ABM1CSErr_flg/1 -> ABM1CSErr/1  "<VHAL_ABM1CSErr_flg>"
  True_VHAL_ABM1CSErr_flg/1 -> ABM1CSErr/2
  [inp_CanValid_bus] -> slr1_1/1
  slr1_1/1 -> ABM1CSErr/3  "<VINP_CANMsgValidABM1_flg>"
  ABM1CSErr/1 -> VINP_ABM1CSErr_flg/1  "VINP_ABM1CSErr_flg"
  ABM1CSErr/2 -> Terminator_1/1
  [BHAL_outputs] -> slr_VHAL_ABM1RCErr_flg/1
  slr_VHAL_ABM1RCErr_flg/1 -> ABM1RCErr/1  "<VHAL_ABM1RCErr_flg>"
  True_VHAL_ABM1RCErr_flg/1 -> ABM1RCErr/2
  [inp_CanValid_bus] -> slr1_2/1
  slr1_2/1 -> ABM1RCErr/3  "<VINP_CANMsgValidABM1_flg>"
  ABM1RCErr/1 -> VINP_ABM1RCErr_flg/1  "VINP_ABM1RCErr_flg"
  ABM1RCErr/2 -> Terminator_2/1
  [BHAL_outputs] -> slr_VHAL_AirBagFailCmd_flg/1
  slr_VHAL_AirBagFailCmd_flg/1 -> AirBagFailCmd/1  "<VHAL_AirBagFailCmd_flg>"
  True_VHAL_AirBagFailCmd_flg/1 -> AirBagFailCmd/2
  [inp_CanValid_bus] -> slr1_3/1
  slr1_3/1 -> AirBagFailCmd/3  "<VINP_CANMsgValidABM1_flg>"
  AirBagFailCmd/1 -> VINP_AirBagFailCmd_flg/1  "VINP_AirBagFailCmd_flg"
  AirBagFailCmd/2 -> Terminator_3/1
  [BHAL_outputs] -> slr_VHAL_ChecksumABM1_enum/1
  slr_VHAL_ChecksumABM1_enum/1 -> ChecksumABM1/1  "<VHAL_ChecksumABM1_enum>"
  True_VHAL_ChecksumABM1_enum/1 -> ChecksumABM1/2
  [inp_CanValid_bus] -> slr1_4/1
  slr1_4/1 -> ChecksumABM1/3  "<VINP_CANMsgValidABM1_flg>"
  ChecksumABM1/1 -> VINP_ChecksumABM1_enum/1  "VINP_ChecksumABM1_enum"
  ChecksumABM1/2 -> Terminator_4/1
  [BHAL_outputs] -> slr_VHAL_CrashOutputSts_enum/1
  slr_VHAL_CrashOutputSts_enum/1 -> CrashOutputSts/1  "<VHAL_CrashOutputSts_enum>"
  True_VHAL_CrashOutputSts_enum/1 -> CrashOutputSts/2
  [inp_CanValid_bus] -> slr1_5/1
  slr1_5/1 -> CrashOutputSts/3  "<VINP_CANMsgValidABM1_flg>"
  CrashOutputSts/1 -> VINP_CrashOutputSts_enum/1  "VINP_CrashOutputSts_enum"
  CrashOutputSts/2 -> Terminator_5/1
  [BHAL_outputs] -> slr_VHAL_DriverSeatBeltCmd_flg/1
  slr_VHAL_DriverSeatBeltCmd_flg/1 -> DriverSeatBeltCmd/1  "<VHAL_DriverSeatBeltCmd_flg>"
  True_VHAL_DriverSeatBeltCmd_flg/1 -> DriverSeatBeltCmd/2
  [inp_CanValid_bus] -> slr1_6/1
  slr1_6/1 -> DriverSeatBeltCmd/3  "<VINP_CANMsgValidABM1_flg>"
  DriverSeatBeltCmd/1 -> VINP_DriverSeatBeltCmd_flg/1  "VINP_DriverSeatBeltCmd_flg"
  DriverSeatBeltCmd/2 -> Terminator_6/1
  [BHAL_outputs] -> slr_VHAL_LifeCountABM1_enum/1
  slr_VHAL_LifeCountABM1_enum/1 -> LifeCountABM1/1  "<VHAL_LifeCountABM1_enum>"
  True_VHAL_LifeCountABM1_enum/1 -> LifeCountABM1/2
  [inp_CanValid_bus] -> slr1_7/1
  slr1_7/1 -> LifeCountABM1/3  "<VINP_CANMsgValidABM1_flg>"
  LifeCountABM1/1 -> VINP_LifeCountABM1_enum/1  "VINP_LifeCountABM1_enum"
  LifeCountABM1/2 -> Terminator_7/1
  [BHAL_outputs] -> slr_VHAL_PsngrSeatBeltCmd_flg/1
  slr_VHAL_PsngrSeatBeltCmd_flg/1 -> PsngrSeatBeltCmd/1  "<VHAL_PsngrSeatBeltCmd_flg>"
  True_VHAL_PsngrSeatBeltCmd_flg/1 -> PsngrSeatBeltCmd/2
  [inp_CanValid_bus] -> slr1_8/1
  slr1_8/1 -> PsngrSeatBeltCmd/3  "<VINP_CANMsgValidABM1_flg>"
  PsngrSeatBeltCmd/1 -> VINP_PsngrSeatBeltCmd_flg/1  "VINP_PsngrSeatBeltCmd_flg"
  PsngrSeatBeltCmd/2 -> Terminator_8/1
  [BHAL_outputs] -> slr_VHAL_RCenterSeatBeltCmd_flg/1
  slr_VHAL_RCenterSeatBeltCmd_flg/1 -> RCenterSeatBeltCmd/1  "<VHAL_RCenterSeatBeltCmd_flg>"
  True_VHAL_RCenterSeatBeltCmd_flg/1 -> RCenterSeatBeltCmd/2
  [inp_CanValid_bus] -> slr1_9/1
  slr1_9/1 -> RCenterSeatBeltCmd/3  "<VINP_CANMsgValidABM1_flg>"
  RCenterSeatBeltCmd/1 -> VINP_RCenterSeatBeltCmd_flg/1  "VINP_RCenterSeatBeltCmd_flg"
  RCenterSeatBeltCmd/2 -> Terminator_9/1
  [BHAL_outputs] -> slr_VHAL_RDriverSeatBeltCmd_flg/1
  slr_VHAL_RDriverSeatBeltCmd_flg/1 -> RDriverSeatBeltCmd/1  "<VHAL_RDriverSeatBeltCmd_flg>"
  True_VHAL_RDriverSeatBeltCmd_flg/1 -> RDriverSeatBeltCmd/2
  [inp_CanValid_bus] -> slr1_10/1
  slr1_10/1 -> RDriverSeatBeltCmd/3  "<VINP_CANMsgValidABM1_flg>"
  RDriverSeatBeltCmd/1 -> VINP_RDriverSeatBeltCmd_flg/1  "VINP_RDriverSeatBeltCmd_flg"
  RDriverSeatBeltCmd/2 -> Terminator_10/1
  [BHAL_outputs] -> slr_VHAL_RPsngrSeatBeltCmd_flg/1
  slr_VHAL_RPsngrSeatBeltCmd_flg/1 -> RPsngrSeatBeltCmd/1  "<VHAL_RPsngrSeatBeltCmd_flg>"
  True_VHAL_RPsngrSeatBeltCmd_flg/1 -> RPsngrSeatBeltCmd/2
  [inp_CanValid_bus] -> slr1_11/1
  slr1_11/1 -> RPsngrSeatBeltCmd/3  "<VINP_CANMsgValidABM1_flg>"
  RPsngrSeatBeltCmd/1 -> VINP_RPsngrSeatBeltCmd_flg/1  "VINP_RPsngrSeatBeltCmd_flg"
  RPsngrSeatBeltCmd/2 -> Terminator_11/1

== system inp/INP/CAN1/SignalCheck/EPAS1 ==
  BHAL_outputs : Inport
  inp_CanValid_bus : Inport  Port=2
  DriIntend : FVT_lib/inp/can_signal_template  SystemSampleTime=-1  VariantActivationTime=update diagram  Latency=0  AutoFrameSizeCalculation=off
      link override defval: Value=KINP_DriIntend_enum_defval
      link override fftdec: Value=KINP_DriIntend_enum_fftdec
      link override fftinc: Value=KINP_DriIntend_enum_fftinc
      link override fftlim: Value=KINP_DriIntend_enum_fftlim
      link override invalid: Value=KINP_DriIntend_enum_invalid
      link override ovrdflg: Value=KINP_DriIntend_enum_ovrdflg
      link override ovrdval: Value=KINP_DriIntend_enum_ovrdval
      link override setvalid: Value=KINP_DriIntend_enum_setvalid
      link override srvcflg: Value=KINP_DriIntend_enum_srvcflg
      link override srvcval: Value=KINP_DriIntend_enum_srvcval
  EPSAOIControl : FVT_lib/inp/can_signal_template  SystemSampleTime=-1  VariantActivationTime=update diagram  Latency=0  AutoFrameSizeCalculation=off
      link override defval: Value=KINP_EPSAOIControl_enum_defval
      link override fftdec: Value=KINP_EPSAOIControl_enum_fftdec
      link override fftinc: Value=KINP_EPSAOIControl_enum_fftinc
      link override fftlim: Value=KINP_EPSAOIControl_enum_fftlim
      link override invalid: Value=KINP_EPSAOIControl_enum_invalid
      link override ovrdflg: Value=KINP_EPSAOIControl_enum_ovrdflg
      link override ovrdval: Value=KINP_EPSAOIControl_enum_ovrdval
      link override setvalid: Value=KINP_EPSAOIControl_enum_setvalid
      link override srvcflg: Value=KINP_EPSAOIControl_enum_srvcflg
      link override srvcval: Value=KINP_EPSAOIControl_enum_srvcval
  Terminator_1 : Terminator
  Terminator_2 : Terminator
  True_VHAL_DriIntend_enum : Constant  Value=TRUE  OutDataTypeStr=boolean
  True_VHAL_EPSAOIControl_enum : Constant  Value=TRUE  OutDataTypeStr=boolean
  slr1_1 : BusSelector  OutputSignals=VINP_CANMsgValidEPAS1_flg
  slr1_2 : BusSelector  OutputSignals=VINP_CANMsgValidEPAS1_flg
  slr_VHAL_DriIntend_enum : BusSelector  OutputSignals=VHAL_DriIntend_enum
  slr_VHAL_EPSAOIControl_enum : BusSelector  OutputSignals=VHAL_EPSAOIControl_enum
  VINP_DriIntend_enum : Outport
  VINP_EPSAOIControl_enum : Outport  Port=2
  wires:
  BHAL_outputs/1 -> [BHAL_outputs]
  inp_CanValid_bus/1 -> [inp_CanValid_bus]
  [BHAL_outputs] -> slr_VHAL_DriIntend_enum/1
  slr_VHAL_DriIntend_enum/1 -> DriIntend/1  "<VHAL_DriIntend_enum>"
  True_VHAL_DriIntend_enum/1 -> DriIntend/2
  [inp_CanValid_bus] -> slr1_1/1
  slr1_1/1 -> DriIntend/3  "<VINP_CANMsgValidEPAS1_flg>"
  DriIntend/1 -> VINP_DriIntend_enum/1  "VINP_DriIntend_enum"
  DriIntend/2 -> Terminator_1/1
  [BHAL_outputs] -> slr_VHAL_EPSAOIControl_enum/1
  slr_VHAL_EPSAOIControl_enum/1 -> EPSAOIControl/1  "<VHAL_EPSAOIControl_enum>"
  True_VHAL_EPSAOIControl_enum/1 -> EPSAOIControl/2
  [inp_CanValid_bus] -> slr1_2/1
  slr1_2/1 -> EPSAOIControl/3  "<VINP_CANMsgValidEPAS1_flg>"
  EPSAOIControl/1 -> VINP_EPSAOIControl_enum/1  "VINP_EPSAOIControl_enum"
  EPSAOIControl/2 -> Terminator_2/1
